simulink model "HW_4_Q1"  (R2023b)
settings: Solver=VariableStepAuto  StartTime=0.0  StopTime=10  RelTol=1e-3
undefined symbols (not defined in the file): A, B, f, fnew, Gu, Gx, gx, H, K, N, Ov, Ox, oy, P, Q, R, ref, v, x0, Y, yc, yx
settings Model: Creator=mani8618  LastModifiedBy=Deven
settings DebuggingCC: UnconnectedInputMsg=warning  UnconnectedOutputMsg=warning  UnconnectedLineMsg=warning
settings ModelReferenceCC: EnableRefExpFcnMdlSchedulingChecks=on
settings RTWCC: DLArmComputeVersion=19.05

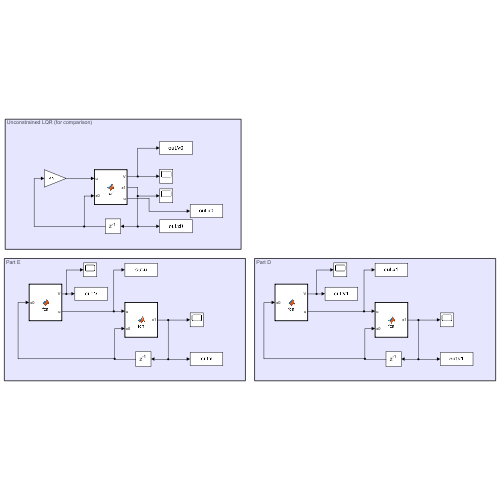
[thumbnail: Simulink's stored preview of the top-level diagram]
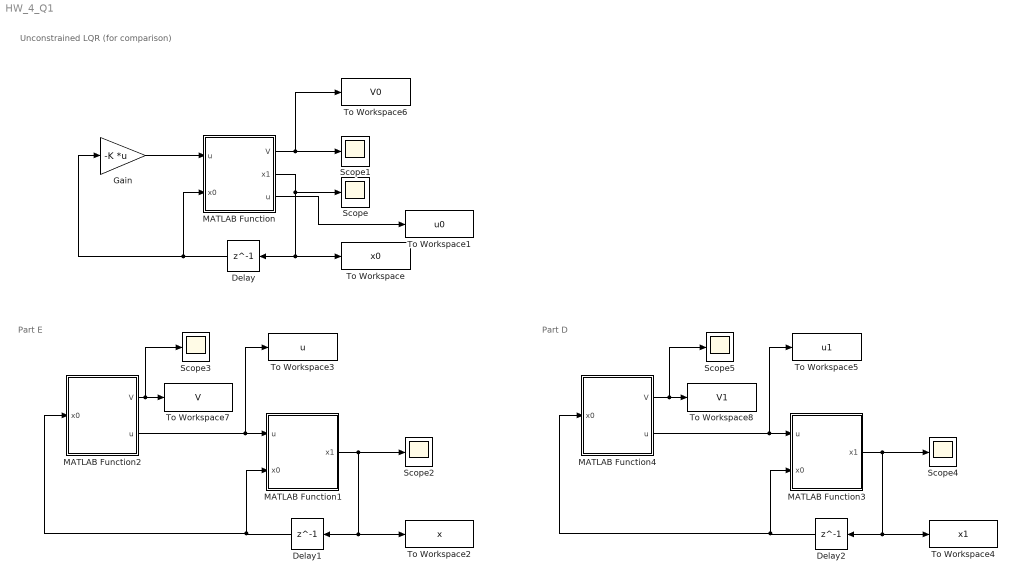
== system HW_4_Q1 ==
  note: Part E
  note: Unconstrained LQR (for comparison)
  note: Part D
  Delay : Delay  DelayLength=1  InitialCondition=x0  SampleTime=.1
  Delay1 : Delay  DelayLength=1  InitialCondition=x0  SampleTime=.1
  Delay2 : Delay  DelayLength=1  InitialCondition=x0  SampleTime=.1
  Gain : Gain  Gain=-K  Multiplication=Matrix(K*u)
  MATLAB Function : MATLAB Function  TreatAsAtomicUnit=on
  MATLAB Function1 : MATLAB Function  TreatAsAtomicUnit=on
  MATLAB Function2 : MATLAB Function  TreatAsAtomicUnit=on
  MATLAB Function3 : MATLAB Function  TreatAsAtomicUnit=on
  MATLAB Function4 : MATLAB Function  TreatAsAtomicUnit=on
  Scope{,1..5} (6 alike) : Scope
  To Workspace : ToWorkspace  VariableName=x0  SampleTime=-1
  To Workspace1 : ToWorkspace  VariableName=u0  SampleTime=-1
  To Workspace2 : ToWorkspace  VariableName=x  SampleTime=-1
  To Workspace3 : ToWorkspace  VariableName=u  SampleTime=-1
  To Workspace4 : ToWorkspace  VariableName=x1  SampleTime=-1
  To Workspace5 : ToWorkspace  VariableName=u1  SampleTime=-1
  To Workspace6 : ToWorkspace  VariableName=V0  SampleTime=-1
  To Workspace7 : ToWorkspace  VariableName=V  SampleTime=-1
  To Workspace8 : ToWorkspace  VariableName=V1  SampleTime=-1
  wires:
  Delay/1 -> Gain/1, MATLAB Function/2(x0)
  Gain/1 -> MATLAB Function/1("u ")
  MATLAB Function/2(x1) -> Delay/1, To Workspace/1, Scope/1
  MATLAB Function/1(V) -> Scope1/1, To Workspace6/1
  Delay1/1 -> MATLAB Function2/1(x0), MATLAB Function1/2(x0)
  MATLAB Function1/1(x1) -> Delay1/1, To Workspace2/1, Scope2/1
  MATLAB Function2/2(u) -> To Workspace3/1, MATLAB Function1/1(u)
  MATLAB Function2/1(V) -> To Workspace7/1, Scope3/1
  MATLAB Function4/1(V) -> Scope5/1, To Workspace8/1
  MATLAB Function4/2(u) -> MATLAB Function3/1(u), To Workspace5/1
  MATLAB Function3/1(x1) -> Scope4/1, To Workspace4/1, Delay2/1
  Delay2/1 -> MATLAB Function3/2(x0), MATLAB Function4/1(x0)
  MATLAB Function/3(u) -> To Workspace1/1

== matlab function HW_4_Q1/MATLAB Function1 ==
  data: u input; x1 output; x0 input; A parameter; B parameter
function x1  = fcn(u,x0,A,B)

x1 = A*x0+B*u;

end

== matlab function HW_4_Q1/MATLAB Function ==
  data: V output; u input; x1 output; x0 input; A parameter; B parameter; P parameter; Gx parameter; Gu parameter; ref parameter; K parameter; u output; R parameter; Q parameter
function [V,x1, u] = fcn(u, x0,A,B,P,Gx, Gu, ref, K, R, Q)

u = Gu*ref + K*Gx*ref + u;
x1 = A*x0+B*u;
V = 0.5*(x0-Gx*ref)'*P*(x0-Gx*ref);

end

== matlab function HW_4_Q1/MATLAB Function2 ==
  data: V output; x0 input; H parameter; u output; f parameter; E parameter; gx parameter; Q parameter; Y parameter; yx parameter; yc parameter; Ox parameter; Ov parameter; oy parameter; v parameter; fnew parameter; Gu parameter; Gx parameter; ref parameter; N parameter; R parameter; P parameter
function [V,u]  = fcn(x0,H,f,E,gx,Q,Y,yx,yc,Ox,Ov,oy, v, fnew, Gu, Gx, ref, N, R, P)
coder.extrinsic('quadprog');
coder.extrinsic('optimoptions');

% z  = f;
z = -fnew*v;
z = quadprog(H,-fnew*v,[Y;Ox],[yc+yx*x0;oy-Ov*v],E,gx*x0,[],[],[],optimoptions('quadprog','Display','none'));
% z = quadprog(H,-fnew*v,[],[],E,gx*x0,[],[],[],optimoptions('quadprog','Display','none'));

V = 1/2*(x0-Gx*ref)'*Q*(x0-Gx*ref)+1/2*z'*H*z-z'*fnew*v+1/2*(N-1)*v'*Gx'*Q*Gx*v+1/2*v'*Gx'*P*Gx*v+1/2*N*v'*Gu'*R*Gu*v;
u = z(1);

end

== matlab function HW_4_Q1/MATLAB Function3 ==
  data: u input; x1 output; x0 input; A parameter; B parameter
function x1  = fcn(u,x0,A,B)

x1 = A*x0+B*u;

end

== matlab function HW_4_Q1/MATLAB Function4 ==
  data: V output; x0 input; H parameter; u output; f parameter; E parameter; gx parameter; Q parameter; Y parameter; yx parameter; yc parameter; Ox parameter; Ov parameter; oy parameter; v parameter; fnew parameter; Gx parameter; Gu parameter; ref parameter; N parameter; P parameter; R parameter
function [V,u]  = fcn(x0,H,f,E,gx,Q,Y,yx,yc,Ox,Ov,oy, v, fnew, Gx, Gu, ref, N, P, R)
coder.extrinsic('quadprog');
coder.extrinsic('optimoptions');

% z  = f;
z = -fnew*v;
% z = quadprog(H,-fnew*v,[Y;Ox],[yc+yx*x0;oy-Ov*v],E,gx*x0,[],[],[],optimoptions('quadprog','Display','none'));
z = quadprog(H,-fnew*v,[],[],E,gx*x0,[],[],[],optimoptions('quadprog','Display','none'));

V = 1/2*(x0-Gx*ref)'*Q*(x0-Gx*ref)+ 1/2*z'*H*z - z'*fnew*v + 1/2*(N-1)*v'*Gx'*Q*Gx*v + 1/2*v'*Gx'*P*Gx*v + 1/2*N*v'*Gu'*R*Gu*v;
u = z(1);

end
